simulink model "Project1_Part1_MODEL"  (R2023b)
settings: Solver=ode1  StartTime=0.0  StopTime=25  FixedStep=0.1  RelTol=1e-3
values from neighbouring files (symbols this model uses):
  A = 100    [Project1_Part1_CODE.m]
  b = b_values(k)    [Project1_Part1_CODE.m]
  F = Frequency_values(f)    [Project1_Part1_CODE.m]
  J = J_values(j)    [Project1_Part1_CODE.m]
  switch_value = S(o)    [Project1_Part1_CODE.m]
  w_0 = w_0_values(i)    [Project1_Part1_CODE.m]
settings Model: Creator=saman  LastModifiedBy=turtl

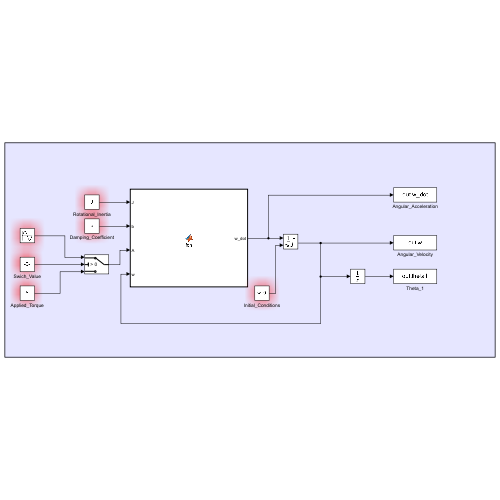
[thumbnail: Simulink's stored preview of the top-level diagram]
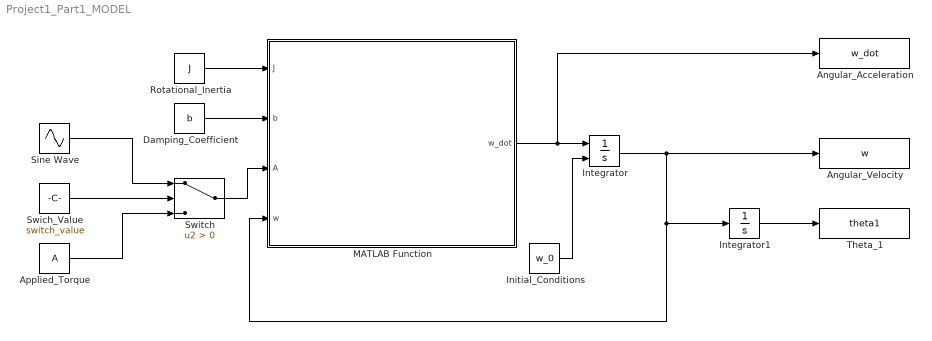
== system Project1_Part1_MODEL ==
  Angular_Acceleration : ToWorkspace  VariableName=w_dot  SaveFormat=Timeseries  SampleTime=-1
  Angular_Velocity : ToWorkspace  VariableName=w  SaveFormat=Timeseries  SampleTime=-1
  Applied_Torque : Constant  Value=A
  Damping_Coefficient : Constant  Value=b
  Initial_Conditions : Constant  Value=w_0
  Integrator : Integrator  InitialConditionSource=external  LimitOutput=on  UpperSaturationLimit=10000  LowerSaturationLimit=0
  Integrator1 : Integrator
  MATLAB Function : MATLAB Function  TreatAsAtomicUnit=on
  Rotational_Inertia : Constant  Value=J
  Sine Wave : Sin  Amplitude=A  Frequency=F  SampleTime=0
  Swich_Value : Constant  Value=switch_value
  Switch : Switch  Criteria=u2 > Threshold  SaturateOnIntegerOverflow=off  InputSameDT=off
  Theta_1 : ToWorkspace  VariableName=theta1  SaveFormat=Timeseries  SampleTime=-1
  wires:
  Rotational_Inertia/1 -> MATLAB Function/1(J)
  Damping_Coefficient/1 -> MATLAB Function/2(b)
  MATLAB Function/1(w_dot) -> Angular_Acceleration/1, Integrator/1
  Initial_Conditions/1 -> Integrator/2
  Integrator/1 -> Angular_Velocity/1, Integrator1/1, MATLAB Function/4(w)
  Integrator1/1 -> Theta_1/1
  Applied_Torque/1 -> Switch/3
  Swich_Value/1 -> Switch/2
  Sine Wave/1 -> Switch/1
  Switch/1 -> MATLAB Function/3(A)

== matlab function Project1_Part1_MODEL/MATLAB Function ==
  data: J input; w_dot output; b input; A input; w input
function w_dot = fcn(J, b, A,w)
w_dot = (1/J)*(A-b*w);
end
